simulink model "mech_motorcycle_stability"  (Simulink 6.0)
settings: Solver=ode45  StartTime=0.0  StopTime=3  RelTol=1e-3  AbsTol=1e-6
PreLoadFcn:
  | vu=53;mech_motorcycle_data
values from neighbouring files (symbols this model uses):
  Cf1 = -13.25+1.302*Zf-(1.39e-4)*Zf^2    [mech_motorcycle_data.m]
  Cf2 = 2.788+0.0165*Zf+(3.9e-6)*Zf^2    [mech_motorcycle_data.m]
  Cf3 = -0.06*Zf    [mech_motorcycle_data.m]
  Cfvf = -300+28.577*Zf-0.0143*Zf^2+(1.431e-6)*Zf^3+(3.347e-10)*Zf^4    [mech_motorcycle_data.m]
  Cfvr = -92.9+23.129*Zr-(4.663/1000)*Zr^2-(6.457e-7)*Zr^3+(1.887e-10)*Zr^4    [mech_motorcycle_data.m]
  Cmvf = -0.281+0.2442*Zf+(8.575e-5)*Zf^2    [mech_motorcycle_data.m]
  Cmvr = 9+0.3573*Zr + (3.378e-5)*Zr^2    [mech_motorcycle_data.m]
  Cr1 = 27.38+0.9727*Zr-(4e-6)*Zr^2    [mech_motorcycle_data.m]
  Cr2 = 2.056+0.01282*Zr+(4.928e-6)*Zr^2    [mech_motorcycle_data.m]
  Cr3 = -0.07*Zr    [mech_motorcycle_data.m]
  G = 9.81    [mech_motorcycle_data.m]
  m = 161    [mech_transmission_data.mat]
  Mfw = 26.5    [mech_motorcycle_data.m]    (also in mech_motorcycle_data_nonlinear.m = 25.6)
  Mp = 0.1    [mech_transmission_data.mat]
  Mrw = 26.5    [mech_motorcycle_data.m]    (also in mech_motorcycle_data_nonlinear.m = 25.6)
  N = 270    [mech_transmission_data.mat]
  Rf = 0.336    [mech_motorcycle_data.m]
  Rr = 0.321    [mech_motorcycle_data.m]
  sigmaf = 0.1012+(1.297e-4)*Zf-(3.267e-8)*Zf^2    [mech_motorcycle_data.m]
  sigmar = 0.03594+(1.941e-4)*Zr-(5.667e-8)*Zr^2+(5.728e-12)*Zr^3    [mech_motorcycle_data.m]
  Zf = ((Mf.value*(bb+kk)+Mr.value*bb+Mb.value*(bb-bb_b)+Mp.value*(bb-bb_p))*G-(vu^2)*(Dc.value*hh_cp+Lc.value*whl_bs/2))/whl_bs    [mech_motorcycle_data.m]
  Zr = (Mf.value+Mr.value+Mp.value+Mb.value)*G-Lc.value*vu^2-Zf    [mech_motorcycle_data.m]
undefined symbols (not defined in the file or in its folder): Crr1, Crr2, D_gamma, D_lamda, D_steer, D_v, D_zita, Dc, ifwy, Ifx, Ifxz, Ifz, Ipx, Ipxz, Ipz, irwx, irwy, Irx, Irxz, iry, Irz, k_gamma, k_lamda, k_steer, k_v, k_zita, Lc, Mb, Mf, Mr, rad, s
libraries: mblibv1 x43, simulink x8, aerospace x2
(part 2 of 2)

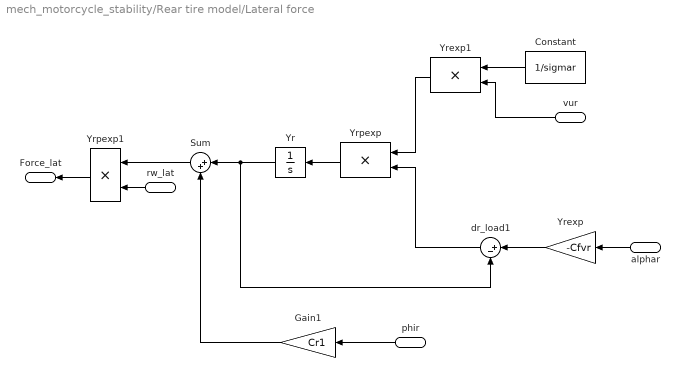
== system mech_motorcycle_stability/Rear tire model/Lateral force ==
  phir : Inport  Orientation=left  Port=1  LatchInput=off
  vur : Inport  Orientation=left  Port=2  LatchInput=off
  alphar : Inport  Orientation=left  Port=3  LatchInput=off
  rw_lat : Inport  Orientation=left  Port=4  LatchInput=off
  Constant : Constant  Orientation=left  Value=1/sigmar
  Gain1 : Gain  Orientation=left  Gain=Cr1  SaturateOnIntegerOverflow=on
  Sum : Sum  Orientation=left  Inputs=|++  SaturateOnIntegerOverflow=on  InputSameDT=on
  Yr : Integrator  Orientation=left  ZeroCross=off
  Yrexp : Gain  Orientation=left  Gain=-Cfvr  SaturateOnIntegerOverflow=on
  Yrexp1 : Product  Orientation=left  SaturateOnIntegerOverflow=on  InputSameDT=on
  Yrpexp : Product  Orientation=left  SaturateOnIntegerOverflow=on  InputSameDT=on
  Yrpexp1 : Product  Orientation=left  SaturateOnIntegerOverflow=on  InputSameDT=on
  dr_load1 : Sum  Orientation=left  Inputs=|+-  SaturateOnIntegerOverflow=on  InputSameDT=on
  Force_lat : Outport  Orientation=left
  wires:
  Yrexp1/1 -> Yrpexp/1
  dr_load1/1 -> Yrpexp/2
  Yrpexp/1 -> Yr/1
  Yr/1 -> dr_load1/2, Sum/1
  vur/1 -> Yrexp1/2
  Yrexp/1 -> dr_load1/1
  alphar/1 -> Yrexp/1
  Constant/1 -> Yrexp1/1
  phir/1 -> Gain1/1
  Gain1/1 -> Sum/2
  Sum/1 -> Yrpexp1/1
  rw_lat/1 -> Yrpexp1/2
  Yrpexp1/1 -> Force_lat/1

== system mech_motorcycle_stability/Rear tire model/Lateral slip computation ==
  drwcp_dt : Inport  Orientation=left  Port=1  LatchInput=off
  rw_lat : Inport  Orientation=left  Port=2  LatchInput=off
  Fcn : Fcn  Orientation=left  Expr=1.0/sqrt(u[1]*u[1] + u[2]*u[2] + u[3]*u[3])
  Product : Product  Orientation=left  SaturateOnIntegerOverflow=on  InputSameDT=on
  Product1 : Product  Orientation=left  Multiplication=Matrix(*)  SaturateOnIntegerOverflow=on  InputSameDT=on
  Reshape : simulink/Math Operations/Reshape  Orientation=left  OutputDimensionality=Row vector  OutputDimensions=[1,1]
  Reshape1 : simulink/Math Operations/Reshape  Orientation=left  OutputDimensionality=Column vector  OutputDimensions=[1,1]
  Trigonometric Function : Trigonometry  Orientation=left  Operator=asin
  alphar : Outport  Orientation=left
  wires:
  Reshape/1 -> Product1/1
  Product1/1 -> Trigonometric Function/1
  Trigonometric Function/1 -> alphar/1
  Reshape1/1 -> Product1/2
  rw_lat/1 -> Reshape1/1
  drwcp_dt/1 -> Product/2, Fcn/1
  Fcn/1 -> Product/1
  Product/1 -> Reshape/1

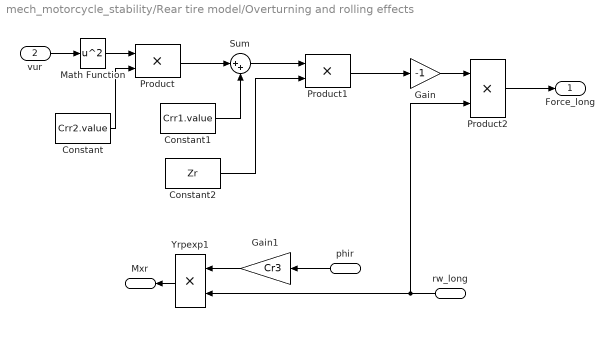
== system mech_motorcycle_stability/Rear tire model/Overturning and rolling effects ==
  rw_long : Inport  Orientation=left  Port=1  LatchInput=off
  vur : Inport  Port=2  LatchInput=off
  phir : Inport  Orientation=left  Port=3  LatchInput=off
  Constant : Constant  Value=Crr2.value
  Constant1 : Constant  Value=Crr1.value
  Constant2 : Constant  Value=Zr
  Gain : Gain  Gain=-1  SaturateOnIntegerOverflow=on
  Gain1 : Gain  Orientation=left  Gain=Cr3  SaturateOnIntegerOverflow=on
  Math Function : Math  Operator=square  SaturateOnIntegerOverflow=on
  Product : Product  SaturateOnIntegerOverflow=on  InputSameDT=on
  Product1 : Product  SaturateOnIntegerOverflow=on  InputSameDT=on
  Product2 : Product  SaturateOnIntegerOverflow=on  InputSameDT=on
  Sum : Sum  Inputs=|++  SaturateOnIntegerOverflow=on  InputSameDT=on
  Yrpexp1 : Product  Orientation=left  SaturateOnIntegerOverflow=on  InputSameDT=on
  Force_long : Outport
  Mxr : Outport  Orientation=left  Port=2
  wires:
  vur/1 -> Math Function/1
  Product/1 -> Sum/1
  Math Function/1 -> Product/1
  Constant/1 -> Product/2
  Constant1/1 -> Sum/2
  Sum/1 -> Product1/1
  Constant2/1 -> Product1/2
  Product1/1 -> Gain/1
  Gain/1 -> Product2/1
  Product2/1 -> Force_long/1
  phir/1 -> Gain1/1
  Gain1/1 -> Yrpexp1/1
  Yrpexp1/1 -> Mxr/1
  rw_long/1 -> Yrpexp1/2, Product2/2

== system mech_motorcycle_stability/Rear tire model/Vertical force ==
  Constant : Constant  Orientation=left  Value=-Zr
  Product2 : Product  Orientation=left  SaturateOnIntegerOverflow=on  InputSameDT=on
  ez : Constant  Orientation=left  Value=[0;0;1]
  Force_vert : Outport  Orientation=left
  wires:
  Product2/1 -> Force_vert/1
  Constant/1 -> Product2/1
  ez/1 -> Product2/2

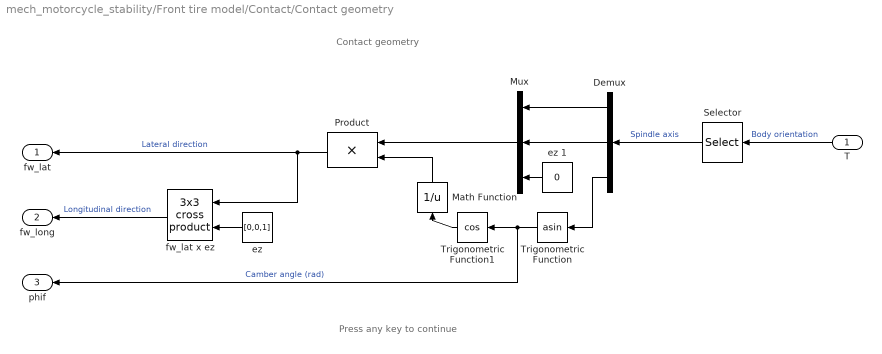
== system mech_motorcycle_stability/Front tire model/Contact/Contact geometry ==
  note: Contact geometry
  note: Press any key to continue
  T : Inport  Orientation=left  Port=1  LatchInput=off
  Demux : Demux  Orientation=left  Outputs=3
  Math Function : Math  Orientation=up  Operator=reciprocal  SaturateOnIntegerOverflow=on
  Mux : Mux  Orientation=left  Inputs=3
  Product : Product  Orientation=left  SaturateOnIntegerOverflow=on  InputSameDT=on
  Selector : Selector  Orientation=left  Elements=[4:6]  InputPortWidth=9
  Trigonometric Function : Trigonometry  Orientation=left  Operator=asin
  Trigonometric Function1 : Trigonometry  Orientation=left  Operator=cos
  "ez " : Constant  Orientation=left  Value=[0,0,1]
  ez 1 : Constant  Orientation=left  Value=0
  fw_lat x ez : aerospace/Axes Transformations/3x3 cross product  Orientation=left
  fw_lat : Outport  Orientation=left
  fw_long : Outport  Orientation=left  Port=2
  phif : Outport  Orientation=left  Port=3
  wires:
  Selector/1 -> Demux/1  "Spindle axis"
  Product/1 -> fw_lat x ez/1, fw_lat/1  "Lateral direction"
  Math Function/1 -> Product/2
  Mux/1 -> Product/1
  Demux/3 -> Trigonometric Function/1
  Trigonometric Function1/1 -> Math Function/1
  Trigonometric Function/1 -> Trigonometric Function1/1, phif/1  "Camber angle (rad)"
  T/1 -> Selector/1  "Body orientation"
  ez 1/1 -> Mux/3
  Demux/2 -> Mux/2
  Demux/1 -> Mux/1
  fw_lat x ez/1 -> fw_long/1  "Longitudinal direction"
  "ez "/1 -> fw_lat x ez/2

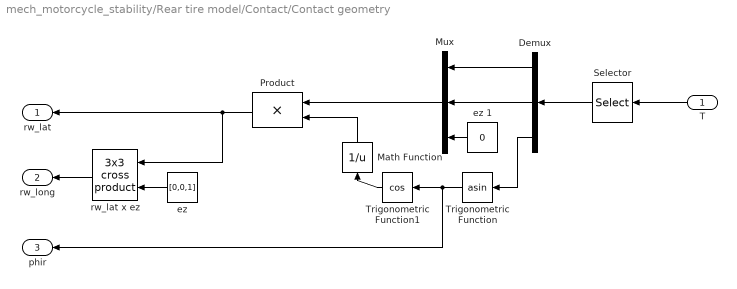
== system mech_motorcycle_stability/Rear tire model/Contact/Contact geometry ==
  T : Inport  Orientation=left  Port=1  LatchInput=off
  Demux : Demux  Orientation=left  Outputs=3
  Math Function : Math  Orientation=up  Operator=reciprocal  SaturateOnIntegerOverflow=on
  Mux : Mux  Orientation=left  Inputs=3
  Product : Product  Orientation=left  SaturateOnIntegerOverflow=on  InputSameDT=on
  Selector : Selector  Orientation=left  Elements=[4:6]  InputPortWidth=9
  Trigonometric Function : Trigonometry  Orientation=left  Operator=asin
  Trigonometric Function1 : Trigonometry  Orientation=left  Operator=cos
  "ez " : Constant  Orientation=left  Value=[0,0,1]
  ez 1 : Constant  Orientation=left  Value=0
  rw_lat x ez : aerospace/Axes Transformations/3x3 cross product  Orientation=left
  rw_lat : Outport  Orientation=left
  rw_long : Outport  Orientation=left  Port=2
  phir : Outport  Orientation=left  Port=3
  wires:
  "ez "/1 -> rw_lat x ez/2
  rw_lat x ez/1 -> rw_long/1
  Demux/1 -> Mux/1
  Demux/2 -> Mux/2
  ez 1/1 -> Mux/3
  T/1 -> Selector/1
  Trigonometric Function/1 -> Trigonometric Function1/1, phir/1
  Trigonometric Function1/1 -> Math Function/1
  Demux/3 -> Trigonometric Function/1
  Mux/1 -> Product/1
  Math Function/1 -> Product/2
  Product/1 -> rw_lat/1, rw_lat x ez/1
  Selector/1 -> Demux/1
